simulink library "fod"  (R2014b)
settings: Solver=ode45  SolverMode=SingleTasking  StartTime=0.0  StopTime=10.0  RelTol=1e-3
libraries: cstblocks x6, fod x3
settings Model: Creator=Alex  LastModifiedBy=Aleksei

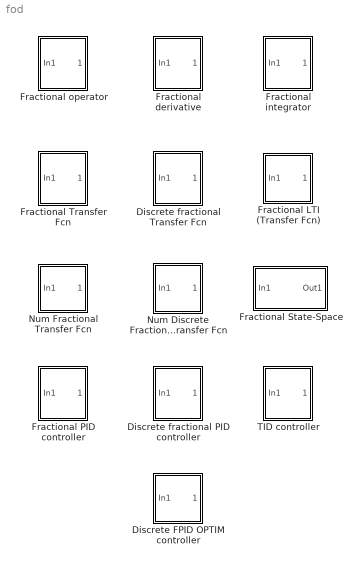
== system fod ==
  Discrete FPID OPTIM controller : Subsystem  mask{fpid_optim_conf=fpid_optim_default_config, dscrMethod=Matched, wc=0, ts=0.001}
      mask prompts: fpid_optim_conf "FPID_OPTIM structure MAT file name"; dscrMethod "Discretization method"; wc "Critical frequency (for Prewarp method)"; ts "Sample time"
      mask init:
      | % Load the MAT file
      | conf = load(fpid_optim_conf);
      | 
      | % Extract required parameters
      | ApproxData = conf.FPID_Optimizer_GUI_config.PlantModel;
      | FPIDParams = conf.FPID_Optimizer_GUI_config.FPIDParams;
      | 
      | % FOPID parameters
      | Kp  = str2num(FPIDParams.Kp);
      | Ki  = str2num(FPIDParams.Ki);
      | lam = str2num(FPIDParams.Lam);
      | Kd  = str2num(FPIDParams.Kd);
      | mu  = str2num(FPIDParams.Mu);
      | 
      | % Approximation details
      | filterTypes   = {'oust', 'ref'};
      | filterToUse   = filterTypes{ApproxData.ApproxType};
      | filterWrange  = str2num(ApproxData.ApproxFreqRange);
      | filterN       = str2num(ApproxData.ApproxOrder);
      | filterZCancel = ApproxData.ZeroCancelation;
      | 
      | % Do the approximation
      | wb=filterWrange(1);
      | wh=filterWrange(2);
      | 
      | % Get controller string
      | [ig1, ig2, str] = fracpid(Kp,Ki,lam,Kd,mu);
      | 
      | % Get the transfer function via OUSTAPID
      | fractf = oustapid(Kp,Ki,lam,Kd,mu,wb,wh,filterN,filterToUse);
      | 
      | if (filterZCancel)
      |     % Make sure that number of poles
      |     % is larger than number of zeros
      |     fractf = toproper(fractf, wh);
      | end
      | 
      | % Discretization type
      | dsctypes = {'zoh', 'foh', 'imp', 'tustin', 'prewarp', 'matched'};
      | dsctype = dsctypes{dscrMethod};
      | if strcmp(dsctype, 'prewarp')
      |     dfraczpk = c2d(fractf, ts, dsctype, wc);
      | else
      |     dfraczpk = c2d(fractf, ts, dsctype);
      | end
      mask TypeOptions dscrMethod: Zero-order hold | Linear interpolation | Impulse-invariant | Bilinear (Tustin) | Prewarp | Matched
      mask Display:
      | port_label('input',1,'');
      | port_label('output', 1, '');
      | disp(['Dsc OPT' char(10) str],'texmode','on');
  Discrete fractional PID controller : Subsystem  mask{Kp=1, Ki=1, lambda=0.5, Kd=1, mu=0.5, freqRange=[0.001; 1000], N=5, useRef=on, dscrMethod=Matched, wc=0, ts=0.5}
      mask prompts: freqRange "Frequency range [wb; wh] [rad/s]"; N "Approximation order"; useRef "Use refined Oustaloup filter"; dscrMethod "Discretization method"; wc "Critical frequency (for Prewarp method)"; ts "Sample time"
      mask init:
      | % Frequency range
      | wb=freqRange(1);
      | wh=freqRange(2);
      | 
      | % Filter type
      | switch useRef
      |     case 0
      |         fMethod = 'oust';
      |     case 1
      |         fMethod = 'ref';
      | end
      | 
      | % Get controller string
      | [ig1, ig2, str] = fracpid(Kp,Ki,lambda,Kd,mu);
      | 
      | % Get the transfer function via OUSTAPID
      | fractf = oustapid(Kp,Ki,lambda,Kd,mu,wb,wh,N,fMethod);
      | 
      | % Make sure that number of poles
      | % is larger than number of zeros
      | fractf = toproper(fractf, wh);
      | 
      | % Discretization type
      | dsctypes = {'zoh', 'foh', 'imp', 'tustin', 'prewarp', 'matched'};
      | dsctype = dsctypes{dscrMethod};
      | if strcmp(dsctype, 'prewarp')
      |     dfraczpk = c2d(fractf, ts, dsctype, wc);
      | else
      |     dfraczpk = c2d(fractf, ts, dsctype);
      | end
      mask TypeOptions dscrMethod: Zero-order hold | Linear interpolation | Impulse-invariant | Bilinear (Tustin) | Prewarp | Matched
      mask Display:
      | port_label('input',1,'');
      | port_label('output', 1, '');
      | disp(['Discrete' char(10) str],'texmode','on');
  Discrete fractional Transfer Fcn : Subsystem  mask(Discrete Fractional Transfer Function){zeroPoly=1, polePoly=s^2.5+1, freqRange=[0.001, 1000], approxNum=5, useRef=off, dscrMethod=Matched, wc=0, ts=0.5}
      mask prompts: zeroPoly "Zero polynomial b(s)"; polePoly "Pole polynomial a(s)"; freqRange "Frequency range [wb, wh] [rad]"; approxNum "Approximation order"; useRef "Use refined Oustaloup filter"; dscrMethod "Discretization method"; wc "Critical frequency (for Prewarp method)"; ts "Sample time"
      mask help: A discrete fractional transfer function system given in continuous form Tf(s)=b(s)/a(s).
      mask init:
      | % Frequency range
      | wb=freqRange(1);
      | wh=freqRange(2);
      | 
      | % Approximation order
      | N = approxNum;
      | 
      | % Filter type
      | switch useRef
      |     case 0
      |         fMethod = 'oust';
      |     case 1
      |         fMethod = 'ref';
      | end
      | 
      | % Get the transfer function
      | fractf = oustapp(newfotf(zeroPoly, polePoly),wb,wh,N,fMethod);
      | 
      | % Discretization type
      | dsctypes = {'zoh', 'foh', 'imp', 'tustin', 'prewarp', 'matched'};
      | dsctype = dsctypes{dscrMethod};
      | 
      | if strcmp(dsctype, 'prewarp')
      |     dfraczpk = c2d(fractf, ts, dsctype, wc);
      | else
      |     dfraczpk = c2d(fractf, ts, dsctype);
      | end
      mask Help: A discrete fractional transfer function system given in continuous form Tf(s)=b(s)/a(s).
      mask TypeOptions dscrMethod: Zero-order hold | Linear interpolation | Impulse-invariant | Bilinear (Tustin) | Prewarp | Matched
      mask Display:
      | port_label('input',1,'');
      | port_label('output', 1, '');
      | disp(['Discrete' char(10) 'Frac Tf(z)']);
  Fractional State-Space : Subsystem  mask(FOSS){A=[-13.0980 -5.8441 5.7893; -5.8441 -16.2606 -5.3504; 5.7893 -5.3504 -7.6497], B=[0 0.4889 -0.3034; 0 1.0347 0; 1.6302 0.7269 -0.7873], C=[0.8884 -1.0689 -2.9443; -1.1471 -0.8095 0], D=[0.3252 1.3703 -0.1022; 0 0 0], q=0.75, iniOff=[0; 0], freqRange=[0.0001 10000], approxNum=5, useRef=off}
      mask prompts: q "Commensurate order q"; iniOff "Initial output offsets"; freqRange "Approximation band"; approxNum "Approximation order"; useRef "Use refined Oustaloup filter"
      mask help: Fractional state-space system
      mask init:
      | % Frequency range
      | wb=freqRange(1);
      | wh=freqRange(2);
      | 
      | % Approximation order
      | N = approxNum;
      | 
      | % Filter type
      | switch useRef
      |     case 0
      |         fMethod = 'oust';
      |     case 1
      |         fMethod = 'ref';
      | end
      | 
      | mySys = foss(A,B,C,D,q);
      | myLtiApprox = zpk(oustapp(mySys,wb,wh,N,fMethod));
      | myLtiApprox = toproper(myLtiApprox, wh);
      mask Help: Fractional state-space system
      mask Display:
      | port_label('input',1,'');
      | port_label('output', 1, '');
      | disp(['D^\alphax=Ax+Bu' char(10) 'y=Cx+Du'], 'TeXMode', 'On');
  Fractional Transfer Fcn : Subsystem  Tag=Fractional Transfer Fcn  Description=Fractional LTI system transfer function  mask(Fractional Transfer Function){zeroPoly=1, polePoly=s^2.5+1, freqRange=[0.001, 1000], approxNum=5, useRef=off}
      mask prompts: zeroPoly "Zero polynomial b(s)"; polePoly "Pole polynomial a(s)"; freqRange "Frequency range [wb, wh]"; approxNum "Approximation order"; useRef "Use refined Oustaloup filter"
      mask help: A fractional transfer function system in form Tf(s)=b(s)/a(s).
      mask init:
      | % Frequency range
      | wb=freqRange(1);
      | wh=freqRange(2);
      | 
      | % Filter
      | T = 1/wh;
      | 
      | % Approximation order
      | N = approxNum;
      | 
      | % Filter type
      | switch useRef
      |     case 0
      |         fMethod = 'oust';
      |     case 1
      |         fMethod = 'ref';
      | end
      | 
      | % Get the transfer function
      | fractf = oustapp(newfotf(zeroPoly, polePoly),wb,wh,N,fMethod);
      mask Help: A fractional transfer function system in form Tf(s)=b(s)/a(s).
      mask Display:
      | port_label('input',1,'');
      | port_label('output', 1, '');
      | disp('Frac Tf(s)', 'texmode' , 'on');
  Fractional derivative : Subsystem  mask(Fractional derivative){gam=0.5, ww=[0.001; 1000], n=5, nFod=off}
      mask prompts: gam "Derivative order"; ww "Frequency range [wb, wh]"; n "Approximation order"; nFod "Use Oustaloup refined filter"
      mask help: Fractional derivative in form s^{gamma}, where gamma is the order of the s operator.
      mask init:
      | % Frequency
      | wb=ww(1);
      | wh=ww(2);
      | 
      | % Filter
      | T = 1/wh;
      | 
      | % Filter type
      | switch nFod
      |     case 0
      |         fMethod = 'oust';
      |     case 1
      |         fMethod = 'ref';
      | end
      | 
      | % Create FOTF object
      | G = newfotf(['s^' num2str(gam)],'1');
      | 
      | % Get Oustaloupe filter
      | G1 = oustapp(G,wb,wh,n,fMethod);
      | 
      | % Make sure that number of poles
      | % is larger than number of zeros
      | s = tf('s');
      | lp_filter = 1/(1+s*(1/wh));
      | 
      | while length(G1.z{1})>length(G1.p{1})
      |    G1 = G1 * lp_filter; 
      | end
      | 
      | % Gamma
      | if isnumeric(gam)
      |     if (gam == 0)
      |         str = '1';
      |     elseif (gam == 1)
      |         str = 'du/dt';
      |     else
      |         str = ['d^{' num2str(gam) '}u/dt^{' num2str(gam) '}'];
      |     end
      | else
      |     str='d^{gam}u/dt';
      | end
      mask Help: Fractional derivative in form s^{gamma}, where gamma is the order of the s operator.
      mask Callback gam:
      | if str2num(get_param(gcb, 'gam')) <= 0
      |     errordlg('Order should be a positive number!', 'Error in operator order');
      |     set_param(gcb, 'gam', '0.5');
      | end
      mask Display:
      | port_label('input',1,'');
      | port_label('output', 1, '');
      | disp(str, 'texmode' , 'on');
  Fractional integrator : Subsystem  mask(Fractional integrator){gam=0.5, ww=[0.001; 1000], n=5, nFod=off}
      mask prompts: gam "Integration order"; ww "Frequency range [wb, wh]"; n "Approximation order"; nFod "Used refined Oustaloup filter"
      mask help: Fractional integrator in form 1/s^{gamma}, where gamma is the order of the s operator.
      mask init:
      | % Frequency
      | wb=ww(1);
      | wh=ww(2);
      | 
      | % Filter
      | T = 1/wh;
      | 
      | % Filter type
      | switch nFod
      |     case 0
      |         fMethod = 'oust';
      |     case 1
      |         fMethod = 'ref';
      | end
      | 
      | % Create FOTF object
      | G = newfotf('1', ['s^' num2str(gam)]);
      | 
      | % Get Oustaloup filter
      | G1 = oustapp(G,wb,wh,n, fMethod);
      | 
      | % Gamma
      | if isnumeric(gam)
      |     if (gam == 0)
      |         str = '1';
      |     elseif (gam == 1)
      |         str = '1/s';
      |     else
      |         str = ['1/s^{' num2str(gam) '}'];
      |     end
      | else
      |     str='1/s^{gam}';
      | end
      mask Help: Fractional integrator in form 1/s^{gamma}, where gamma is the order of the s operator.
      mask Callback gam:
      | if str2num(get_param(gcb, 'gam')) <= 0
      |     errordlg('Order should be a positive number!', 'Error in operator order');
      |     set_param(gcb, 'gam', '0.5');
      | end
      mask Callback n:
      | if str2num(get_param(gcb, 'gam')) < 0
      |     errordlg('Order should be a positive number!', 'Error in operator order');
      |     set_param(gcb, 'gam', '0.5');
      | end
      mask Display:
      | port_label('input',1,'');
      | port_label('output', 1, '');
      | disp(str, 'texmode' , 'on');
  Fractional operator : Subsystem  Tag=Fractional operator  mask(Fractional operator){K=1, gam=0.25, ww=[0.001, 1000], n=5}
      mask prompts: K "Gain"; gam "Order in range (-1; 1)"; ww "Frequency range [wb, wh]"; n "Approximation order"
      mask help: Fractional operator in form K*s^{gamma}, where K is the gain and gamma is the order of the s operator.
      mask init:
      | wb=ww(1);
      | wh=ww(2);
      | G1=new_fod(gam,n,wb,wh,10,9);
      | G=tf(G1);
      | num=G.num{1};
      | den=G.den{1};
      | T=1/wh;
      | 
      | % Gain dot
      | if gam ~= 0
      |     dotAdd = '\cdot';
      | else
      |     dotAdd = '';
      | end
      | 
      | % Gain
      | if isnumeric(K)
      |     if (K == -1)
      |         str = '-';
      |     elseif (K == 1)
      |         str = '';
      |     else
      |         str = [num2str(K) dotAdd];
      |     end
      | else
      |     str = ['K' dotAdd];
      | end
      | 
      | % Gamma
      | if isnumeric(gam)
      |     if (gam < 0)
      |         if (gam == -1)
      |             sstr = '1/s';
      |         else
      |             sstr = ['1/{s^{' num2str(abs(gam)) '}}'];
      |         end
      |     elseif (gam == 0)
      |         if isnumeric(K)
      |             if K == -1 || K == 1
      |                 sstr = '1';
      |             else
      |                 sstr = '';
      |             end
      |         else
      |             sstr = '';
      |         end
      |     elseif (gam == 1)
      |         sstr = 's';
      |     else
      |         sstr = ['s^{' num2str(gam) '}'];
      |     end
      | else
      |     sstr=[str 's^{gam}'];
      | end
      | 
      | str = [str sstr];
      mask Help: Fractional operator in form K*s^{gamma}, where K is the gain and gamma is the order of the s operator.
      mask Callback gam:
      | if abs(str2num(get_param(gcb, 'gam'))) >= 1
      |     errordlg('Order should be in range (-1; 1)', 'Error in operator order');
      |     set_param(gcb, 'gam', '0.5');
      | end
      mask Display:
      | port_label('input',1,'');
      | port_label('output', 1, '');
      | disp(str, 'texmode' , 'on');
  Fractional LTI (Transfer Fcn) : Subsystem  mask(Fractional LTI System){G=fotf('s'), freqRange=[0.001 1000], approxNum=5, useRef=off}
      mask prompts: G "LTI system variable"; freqRange "Approximation frequency range [wb, wh]"; approxNum "Approximation order N"; useRef "Use refined Oustaloup filter"
      mask help: A fractional LTI system.
      mask init:
      | % Frequency range
      | wb=freqRange(1);
      | wh=freqRange(2);
      | 
      | % Approximation order
      | N = approxNum;
      | 
      | % Filter
      | T = 1/wh;
      | 
      | % Filter type
      | switch useRef
      |     case 0
      |         fMethod = 'oust';
      |     case 1
      |         fMethod = 'ref';
      | end
      | 
      | % Get the LTI system from base workspace (as transfer function)
      | sys = evalin('base', G);
      | fractf = zpk(oustapp(sys,wb,wh,N,fMethod));
      | fractf = toproper(fractf, wh);
      mask Help: A fractional LTI system.
      mask Display:
      | port_label('input',1,'');
      | port_label('output', 1, '');
      | disp(G);
  Fractional PID controller : Subsystem  mask(Fractional PID){Kp=1, Ki=1, lambda=0.5, Kd=1, mic=0.5, freqRange=[0.001, 1000], N=5}
      mask prompts: mic "mu"; freqRange "Frequency range [wb, wh]"; N "Approximation order"
      mask help:
      | Fractional PID with parameters Kp, Ki, Kd and extended parameters lambda and delta:
      |
      | PI^{lambda}D^{mu} = Kp + Ki*s^-{lambda} + Kd*s^{mu}
      mask init:
      | wb = freqRange(1);
      | wh = freqRange(2);
      | 
      | T = 1/wh;
      | 
      | [p_,c_,str]=fracpid(Kp,Ki,lambda,Kd,mic);
      mask Help:
      | Fractional PID with parameters Kp, Ki, Kd and extended parameters lambda and delta:
      | 
      | PI^{lambda}D^{mu} = Kp + Ki*s^-{lambda} + Kd*s^{mu}
      mask Display:
      | port_label('input',1,'');
      | port_label('output', 1, '');
      | disp(str, 'texmode' , 'on');
  Num Discrete Fractional Transfer Fcn : Subsystem  mask(Discrete Fractional Transfer Function (numerical polynomial coefficient/exponents)){b=[1], nb=[0], a=[1 1], na=[0.5 0], freqRange=[0.001, 1000], approxNum=5, useRef=off, dscrMethod=Matched, wc=0, ts=0.001}
      mask prompts: b "Zero polynomial coefficients:"; nb "Zero polynomial exponents:"; a "Pole polynomial coefficients:"; na "Pole polynomial exponents:"; freqRange "Frequency range [wb, wh]"; approxNum "Approximation order"; useRef "Use refined Oustaloup filter"; dscrMethod "Discretization method"; wc "Critical frequency (for Prewarp method)"; ts "Sample time Ts:"
      mask help:
      | A discrete fractional transfer function system given in continuous form
      | Tf(s)=b(s)/a(s). This block allows to use numerical (vector) entry of
      | coefficients/exponents.
      mask init:
      | % Frequency range
      | wb=freqRange(1);
      | wh=freqRange(2);
      | 
      | % Approximation order
      | N = approxNum;
      | 
      | % Filter type
      | switch useRef
      |     case 0
      |         fMethod = 'oust';
      |     case 1
      |         fMethod = 'ref';
      | end
      | 
      | % Get the transfer function
      | fractf = oustapp(fotf(a,na,b,nb),wb,wh,N,fMethod);
      | 
      | % Discretization type
      | dsctypes = {'zoh', 'foh', 'imp', 'tustin', 'prewarp', 'matched'};
      | dsctype = dsctypes{dscrMethod};
      | 
      | if strcmp(dsctype, 'prewarp')
      |     dfraczpk = c2d(fractf, ts, dsctype, wc);
      | else
      |     dfraczpk = c2d(fractf, ts, dsctype);
      | end
      mask Help:
      | A discrete fractional transfer function system given in continuous form
      | Tf(s)=b(s)/a(s). This block allows to use numerical (vector) entry of
      | coefficients/exponents.
      mask TypeOptions dscrMethod: Zero-order hold | Linear interpolation | Impulse-invariant | Bilinear (Tustin) | Prewarp | Matched
      mask Display:
      | port_label('input',1,'');
      | port_label('output', 1, '');
      | disp(['Discrete' char(10) 'Num Fr Tf']);
  Num Fractional Transfer Fcn : Subsystem  mask(Fractional Transfer Function (numerical polynomial coefficient/exponents)){b=[1], nb=[0], a=[1 1], na=[0.5 0], freqRange=[0.001, 1000], approxNum=5, useRef=off}
      mask prompts: b "Zero polynomial coefficients:"; nb "Zero polynomial exponents:"; a "Pole polynomial coefficients:"; na "Pole polynomial exponents:"; freqRange "Frequency range [wb, wh]"; approxNum "Approximation order N"; useRef "Use refined Oustaloup filter"
      mask help:
      | A fractional transfer function system in form Tf(s)=b(s)/a(s). This block
      | allows to use numerical (vector) entry of coefficients/exponents.
      mask init:
      | % Frequency range
      | wb=freqRange(1);
      | wh=freqRange(2);
      | 
      | % Filter
      | T = 1/wh;
      | 
      | % Approximation order
      | N = approxNum;
      | 
      | % Filter type
      | switch useRef
      |     case 0
      |         fMethod = 'oust';
      |     case 1
      |         fMethod = 'ref';
      | end
      | 
      | % Get the transfer function
      | fractf = oustapp(fotf(a,na,b,nb),wb,wh,N,fMethod);
      mask Help:
      | A fractional transfer function system in form Tf(s)=b(s)/a(s). This block
      | allows to use numerical (vector) entry of coefficients/exponents.
      mask Display:
      | port_label('input',1,'');
      | port_label('output', 1, '');
      | disp('Num Fr Tf', 'texmode' , 'on');
  TID controller : Subsystem  mask{Kt=1, K_n=3, Ki=1, Kd=1, freqRange=[0.001, 1000], N=5}
      mask prompts: K_n "n (for s^-1/n)"; freqRange "Frequency range [wb, wh]"; N "Approximation order"
      mask init:
      | wb = freqRange(1);
      | wh = freqRange(2);
      mask Display:
      | port_label('input',1,'');
      | port_label('output', 1, '');
      | disp('TID', 'texmode' , 'on');

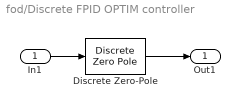
== system fod/Discrete FPID OPTIM controller ==
  In1 : Inport
  Discrete Zero-Pole : DiscreteZeroPole  Zeros=dfraczpk.z{1}  Poles=dfraczpk.p{1}  Gain=dfraczpk.k  SampleTime=ts
  Out1 : Outport
  wires:
  In1/1 -> Discrete Zero-Pole/1
  Discrete Zero-Pole/1 -> Out1/1

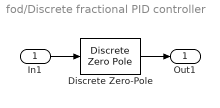
== system fod/Discrete fractional PID controller ==
  In1 : Inport
  Discrete Zero-Pole : DiscreteZeroPole  Zeros=dfraczpk.z{1}  Poles=dfraczpk.p{1}  Gain=dfraczpk.k  SampleTime=ts
  Out1 : Outport
  wires:
  In1/1 -> Discrete Zero-Pole/1
  Discrete Zero-Pole/1 -> Out1/1

== system fod/Discrete fractional Transfer Fcn ==
  In1 : Inport
  Discrete Zero-Pole : DiscreteZeroPole  Zeros=dfraczpk.z{1}  Poles=dfraczpk.p{1}  Gain=dfraczpk.k  SampleTime=ts
  Out1 : Outport
  wires:
  In1/1 -> Discrete Zero-Pole/1
  Discrete Zero-Pole/1 -> Out1/1

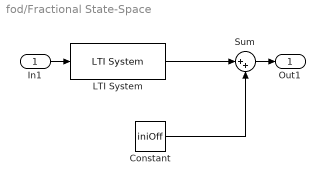
== system fod/Fractional State-Space ==
  In1 : Inport
  Constant : Constant  Value=iniOff
  LTI System : cstblocks/LTI System  sys=myLtiApprox  IC=[]
  Sum : Sum  Inputs=|++
  Out1 : Outport
  wires:
  Constant/1 -> Sum/2
  In1/1 -> LTI System/1
  Sum/1 -> Out1/1
  LTI System/1 -> Sum/1

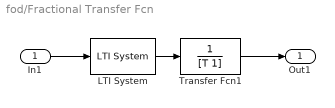
== system fod/Fractional Transfer Fcn ==
  In1 : Inport
  LTI System : cstblocks/LTI System  sys=fractf  IC=[]
  Transfer Fcn1 : TransferFcn  Denominator=[T 1]
  Out1 : Outport
  wires:
  In1/1 -> LTI System/1
  LTI System/1 -> Transfer Fcn1/1
  Transfer Fcn1/1 -> Out1/1

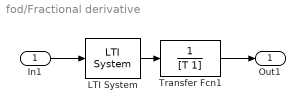
== system fod/Fractional derivative ==
  In1 : Inport
  LTI System : cstblocks/LTI System  sys=G1  IC=[]
  Transfer Fcn1 : TransferFcn  Denominator=[T 1]
  Out1 : Outport
  wires:
  In1/1 -> LTI System/1
  LTI System/1 -> Transfer Fcn1/1
  Transfer Fcn1/1 -> Out1/1

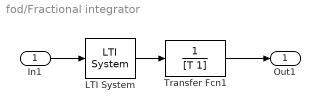
== system fod/Fractional integrator ==
  In1 : Inport
  LTI System : cstblocks/LTI System  sys=G1  IC=[]
  Transfer Fcn1 : TransferFcn  Denominator=[T 1]
  Out1 : Outport
  wires:
  In1/1 -> LTI System/1
  LTI System/1 -> Transfer Fcn1/1
  Transfer Fcn1/1 -> Out1/1

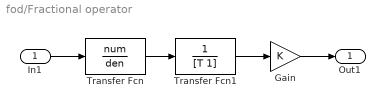
== system fod/Fractional operator ==
  In1 : Inport
  Gain : Gain  Gain=K
  Transfer Fcn : TransferFcn  Numerator=num  Denominator=den
  Transfer Fcn1 : TransferFcn  Denominator=[T 1]
  Out1 : Outport
  wires:
  Transfer Fcn/1 -> Transfer Fcn1/1
  In1/1 -> Transfer Fcn/1
  Transfer Fcn1/1 -> Gain/1
  Gain/1 -> Out1/1

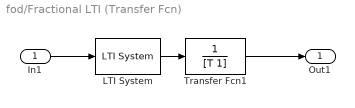
== system fod/Fractional LTI (Transfer Fcn) ==
  In1 : Inport
  LTI System : cstblocks/LTI System  sys=fractf  IC=[]
  Transfer Fcn1 : TransferFcn  Denominator=[T 1]
  Out1 : Outport
  wires:
  In1/1 -> LTI System/1
  LTI System/1 -> Transfer Fcn1/1
  Transfer Fcn1/1 -> Out1/1

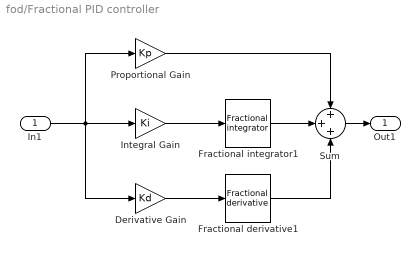
== system fod/Fractional PID controller ==
  In1 : Inport
  Derivative Gain : Gain  Gain=Kd
  Fractional derivative1 : fod/Fractional derivative  gam=mic  ww=[wb; wh]  n=N  nFod=off
  Fractional integrator1 : fod/Fractional integrator  gam=lambda  ww=[wb; wh]  n=N  nFod=off
  Integral Gain : Gain  Gain=Ki
  Proportional Gain : Gain  Gain=Kp
  Sum : Sum  Inputs=+++  SaturateOnIntegerOverflow=on  InputSameDT=on  OutDataTypeStr=Inherit: Same as first input
  Out1 : Outport
  wires:
  Integral Gain/1 -> Fractional integrator1/1
  Proportional Gain/1 -> Sum/1
  Fractional integrator1/1 -> Sum/2
  Fractional derivative1/1 -> Sum/3
  Derivative Gain/1 -> Fractional derivative1/1
  In1/1 -> Integral Gain/1, Proportional Gain/1, Derivative Gain/1
  Sum/1 -> Out1/1

== system fod/Num Discrete Fractional Transfer Fcn ==
  In1 : Inport
  Discrete Zero-Pole : DiscreteZeroPole  Zeros=dfraczpk.z{1}  Poles=dfraczpk.p{1}  Gain=dfraczpk.k  SampleTime=ts
  Out1 : Outport
  wires:
  In1/1 -> Discrete Zero-Pole/1
  Discrete Zero-Pole/1 -> Out1/1

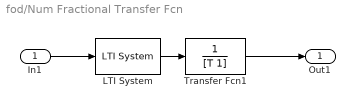
== system fod/Num Fractional Transfer Fcn ==
  In1 : Inport
  LTI System : cstblocks/LTI System  sys=fractf  IC=[]
  Transfer Fcn1 : TransferFcn  Denominator=[T 1]
  Out1 : Outport
  wires:
  Transfer Fcn1/1 -> Out1/1
  LTI System/1 -> Transfer Fcn1/1
  In1/1 -> LTI System/1

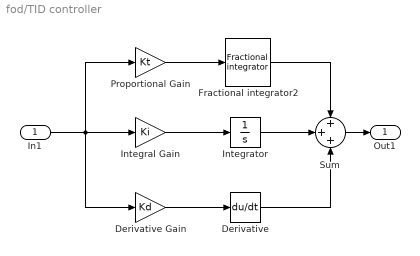
== system fod/TID controller ==
  In1 : Inport
  Derivative : Derivative
  Derivative Gain : Gain  Gain=Kd
  Fractional integrator2 : fod/Fractional integrator  gam=1/K_n  ww=[wb; wh]  n=N  nFod=on
  Integral Gain : Gain  Gain=Ki
  Integrator : Integrator
  Proportional Gain : Gain  Gain=Kt
  Sum : Sum  Inputs=+++  SaturateOnIntegerOverflow=on  InputSameDT=on  OutDataTypeStr=Inherit: Same as first input
  Out1 : Outport
  wires:
  Integral Gain/1 -> Integrator/1
  Proportional Gain/1 -> Fractional integrator2/1
  Integrator/1 -> Sum/2
  Derivative/1 -> Sum/3
  Derivative Gain/1 -> Derivative/1
  In1/1 -> Integral Gain/1, Proportional Gain/1, Derivative Gain/1
  Sum/1 -> Out1/1
  Fractional integrator2/1 -> Sum/1
